simulink model "untitled"  (R2022a)
settings: Solver=FixedStepDiscrete  StartTime=0.0  StopTime=10.0  RelTol=1e-3
libraries: simulink x7
settings Model: DataDictionary=test.sldd  Creator=15801  LastModifiedBy=JSF
settings OptimizationCC: DefaultParameterBehavior=Inlined  EnhancedBackFolding=on  PassReuseOutputArgsAs=Individual arguments  ZeroExternalMemoryAtStartup=off  ZeroInternalMemoryAtStartup=off  OptimizeBlockOrder=speed  DifferentSizesBufferReuse=on  OptimizationCustomize=off  EfficientTunableParamExpr=on
settings DebuggingCC: ParameterTunabilityLossMsg=error
settings ModelReferenceCC: EnableRefExpFcnMdlSchedulingChecks=off
settings SFSimCC: MATLABDynamicMemAlloc=off
settings RTWCC: SystemTargetFile=ert.tlc  TemplateMakefile=ert_default_tmf
settings CodeAppCC: ForceParamTrailComments=on  IgnoreCustomStorageClasses=off  OperatorAnnotations=on  SimulinkDataObjDesc=on  SFDataObjDesc=on  InsertBlockDesc=on
settings ERTTargetCC: TargetLangStandard=C99 (ISO)  GenerateSampleERTMain=on  InlinedParameterPlacement=NonHierarchical  ERTCustomFileTemplate=example_file_process.tlc

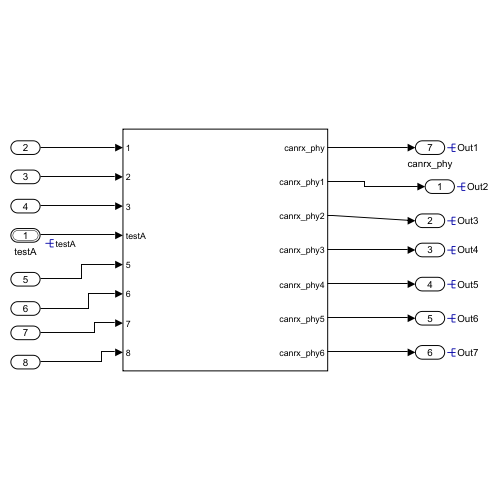
[thumbnail: Simulink's stored preview of the top-level diagram]
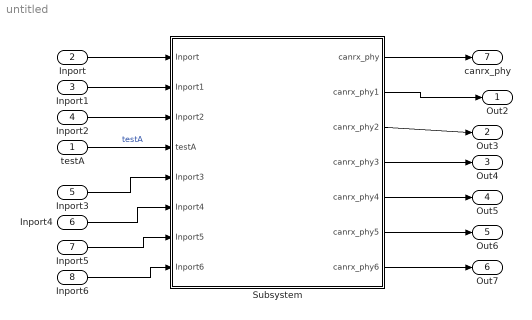
== system untitled ==
  testA : Inport  OutDataTypeStr=Bus: test
  Inport : Inport  Port=2
  Inport1 : Inport  Port=3
  Inport2 : Inport  Port=4
  Inport3 : Inport  Port=5
  Inport4 : Inport  Port=6
  Inport5 : Inport  Port=7
  Inport6 : Inport  Port=8
  Subsystem : Subsystem
  Out2 : Outport  SignalName=Out2
      settings: MustResolveToSignalObject=on
  Out3 : Outport  Port=2  SignalName=Out3
      settings: MustResolveToSignalObject=on
  Out4 : Outport  Port=3  SignalName=Out4
      settings: MustResolveToSignalObject=on
  Out5 : Outport  Port=4  SignalName=Out5
      settings: MustResolveToSignalObject=on
  Out6 : Outport  Port=5  SignalName=Out6
      settings: MustResolveToSignalObject=on
  Out7 : Outport  Port=6  SignalName=Out7
      settings: MustResolveToSignalObject=on
  canrx_phy : Outport  Port=7  SignalName=Out1
      settings: MustResolveToSignalObject=on
  wires:
  Subsystem/5(canrx_phy4) -> Out5/1
  Inport/1 -> Subsystem/1(Inport)
  Inport1/1 -> Subsystem/2(Inport1)
  Inport6/1 -> Subsystem/8(Inport6)
  testA/1 -> Subsystem/4(testA)  "testA"
  Inport3/1 -> Subsystem/5(Inport3)
  Inport2/1 -> Subsystem/3(Inport2)
  Inport4/1 -> Subsystem/6(Inport4)
  Inport5/1 -> Subsystem/7(Inport5)
  Subsystem/1(canrx_phy) -> canrx_phy/1
  Subsystem/2(canrx_phy1) -> Out2/1
  Subsystem/3(canrx_phy2) -> Out3/1
  Subsystem/4(canrx_phy3) -> Out4/1
  Subsystem/6(canrx_phy5) -> Out6/1
  Subsystem/7(canrx_phy6) -> Out7/1

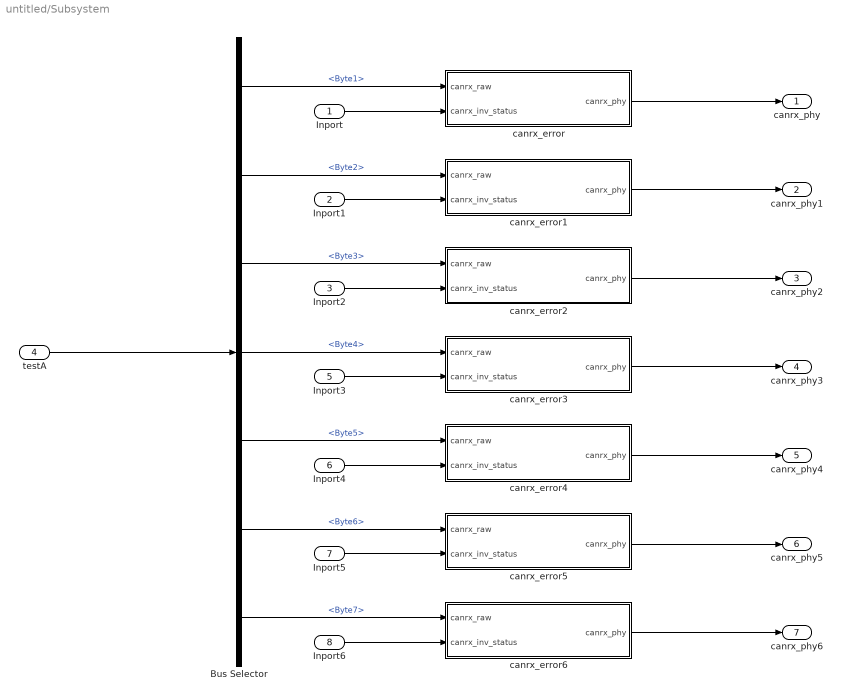
== system untitled/Subsystem ==
  Inport : Inport
  Inport1 : Inport  Port=2
  Inport2 : Inport  Port=3
  testA : Inport  Port=4
  Inport3 : Inport  Port=5
  Inport4 : Inport  Port=6
  Inport5 : Inport  Port=7
  Inport6 : Inport  Port=8
  Bus Selector : BusSelector  OutputSignals=Byte1,Byte2,Byte3,Byte4,Byte5,Byte6,Byte7
  canrx_error : Subsystem  TreatAsAtomicUnit=on
  canrx_error1 : Subsystem  TreatAsAtomicUnit=on
  canrx_error2 : Subsystem  TreatAsAtomicUnit=on
  canrx_error3 : Subsystem  TreatAsAtomicUnit=on
  canrx_error4 : Subsystem  TreatAsAtomicUnit=on
  canrx_error5 : Subsystem  TreatAsAtomicUnit=on
  canrx_error6 : Subsystem  TreatAsAtomicUnit=on
  canrx_phy : Outport
  canrx_phy1 : Outport  Port=2
  canrx_phy2 : Outport  Port=3
  canrx_phy3 : Outport  Port=4
  canrx_phy4 : Outport  Port=5
  canrx_phy5 : Outport  Port=6
  canrx_phy6 : Outport  Port=7
  wires:
  Bus Selector/1 -> canrx_error/1(canrx_raw)  "<Byte1>"
  Bus Selector/2 -> canrx_error1/1(canrx_raw)  "<Byte2>"
  Inport1/1 -> canrx_error1/2(canrx_inv_status)
  Inport/1 -> canrx_error/2(canrx_inv_status)
  Inport6/1 -> canrx_error6/2(canrx_inv_status)
  Bus Selector/7 -> canrx_error6/1(canrx_raw)  "<Byte7>"
  Bus Selector/6 -> canrx_error5/1(canrx_raw)  "<Byte6>"
  Inport2/1 -> canrx_error2/2(canrx_inv_status)
  canrx_error5/1(canrx_phy) -> canrx_phy5/1
  Inport5/1 -> canrx_error5/2(canrx_inv_status)
  Bus Selector/3 -> canrx_error2/1(canrx_raw)  "<Byte3>"
  Bus Selector/5 -> canrx_error4/1(canrx_raw)  "<Byte5>"
  Bus Selector/4 -> canrx_error3/1(canrx_raw)  "<Byte4>"
  Inport3/1 -> canrx_error3/2(canrx_inv_status)
  Inport4/1 -> canrx_error4/2(canrx_inv_status)
  canrx_error6/1(canrx_phy) -> canrx_phy6/1
  testA/1 -> Bus Selector/1
  canrx_error3/1(canrx_phy) -> canrx_phy3/1
  canrx_error/1(canrx_phy) -> canrx_phy/1
  canrx_error4/1(canrx_phy) -> canrx_phy4/1
  canrx_error1/1(canrx_phy) -> canrx_phy1/1
  canrx_error2/1(canrx_phy) -> canrx_phy2/1

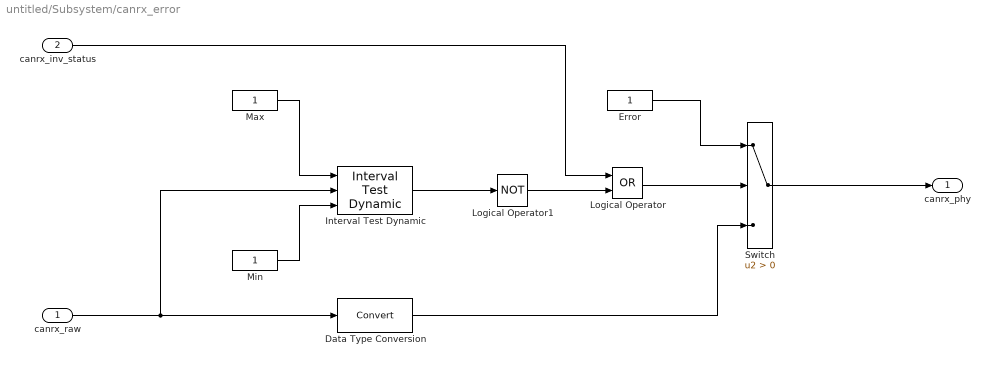
== system untitled/Subsystem/canrx_error ==
  canrx_raw : Inport
  canrx_inv_status : Inport  Port=2
  Data Type Conversion : DataTypeConversion  SaturateOnIntegerOverflow=off  RndMeth=Floor
  Error : Constant  OutDataTypeStr=Inherit: Inherit via back propagation
  Interval Test Dynamic : simulink/Logic and Bit Operations/Interval Test Dynamic  IntervalClosedRight=on  IntervalClosedLeft=on  OutDataTypeStr=boolean
  Logical Operator : Logic  Operator=OR  AllPortsSameDT=off  OutDataTypeStr=boolean
  Logical Operator1 : Logic  Operator=NOT  AllPortsSameDT=off  OutDataTypeStr=boolean
  Max : Constant  OutDataTypeStr=Inherit: Inherit via back propagation
  Min : Constant  OutDataTypeStr=Inherit: Inherit via back propagation
  Switch : Switch  Criteria=u2 > Threshold  SaturateOnIntegerOverflow=off  InputSameDT=off
  canrx_phy : Outport
  wires:
  canrx_raw/1 -> Data Type Conversion/1, Interval Test Dynamic/2
  Max/1 -> Interval Test Dynamic/1
  Min/1 -> Interval Test Dynamic/3
  Data Type Conversion/1 -> Switch/3
  Interval Test Dynamic/1 -> Logical Operator1/1
  Logical Operator1/1 -> Logical Operator/2
  canrx_inv_status/1 -> Logical Operator/1
  Logical Operator/1 -> Switch/2
  Error/1 -> Switch/1
  Switch/1 -> canrx_phy/1

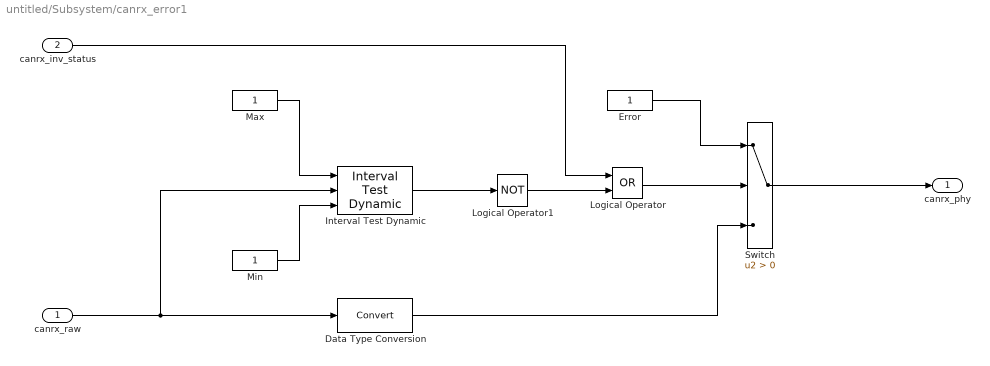
== system untitled/Subsystem/canrx_error1 ==
  canrx_raw : Inport
  canrx_inv_status : Inport  Port=2
  Data Type Conversion : DataTypeConversion  SaturateOnIntegerOverflow=off  RndMeth=Floor
  Error : Constant  OutDataTypeStr=Inherit: Inherit via back propagation
  Interval Test Dynamic : simulink/Logic and Bit Operations/Interval Test Dynamic  IntervalClosedRight=on  IntervalClosedLeft=on  OutDataTypeStr=boolean
  Logical Operator : Logic  Operator=OR  AllPortsSameDT=off  OutDataTypeStr=boolean
  Logical Operator1 : Logic  Operator=NOT  AllPortsSameDT=off  OutDataTypeStr=boolean
  Max : Constant  OutDataTypeStr=Inherit: Inherit via back propagation
  Min : Constant  OutDataTypeStr=Inherit: Inherit via back propagation
  Switch : Switch  Criteria=u2 > Threshold  SaturateOnIntegerOverflow=off  InputSameDT=off
  canrx_phy : Outport
  wires:
  canrx_raw/1 -> Data Type Conversion/1, Interval Test Dynamic/2
  Max/1 -> Interval Test Dynamic/1
  Min/1 -> Interval Test Dynamic/3
  Data Type Conversion/1 -> Switch/3
  Interval Test Dynamic/1 -> Logical Operator1/1
  Logical Operator1/1 -> Logical Operator/2
  canrx_inv_status/1 -> Logical Operator/1
  Logical Operator/1 -> Switch/2
  Error/1 -> Switch/1
  Switch/1 -> canrx_phy/1

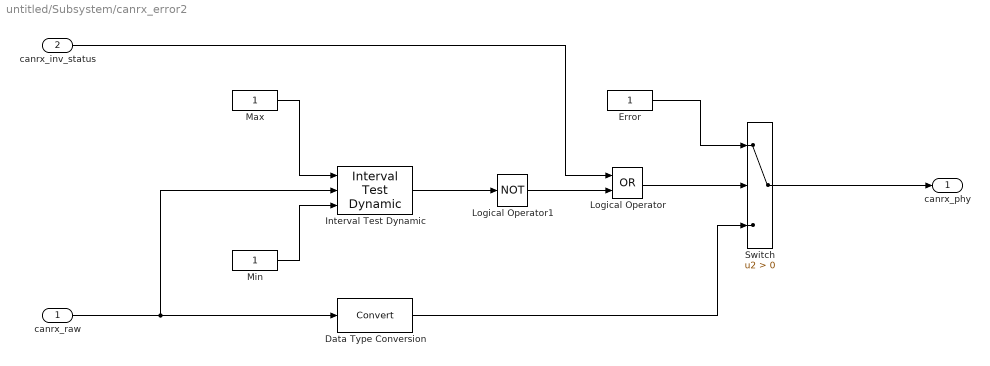
== system untitled/Subsystem/canrx_error2 ==
  canrx_raw : Inport
  canrx_inv_status : Inport  Port=2
  Data Type Conversion : DataTypeConversion  SaturateOnIntegerOverflow=off  RndMeth=Floor
  Error : Constant  OutDataTypeStr=Inherit: Inherit via back propagation
  Interval Test Dynamic : simulink/Logic and Bit Operations/Interval Test Dynamic  IntervalClosedRight=on  IntervalClosedLeft=on  OutDataTypeStr=boolean
  Logical Operator : Logic  Operator=OR  AllPortsSameDT=off  OutDataTypeStr=boolean
  Logical Operator1 : Logic  Operator=NOT  AllPortsSameDT=off  OutDataTypeStr=boolean
  Max : Constant  OutDataTypeStr=Inherit: Inherit via back propagation
  Min : Constant  OutDataTypeStr=Inherit: Inherit via back propagation
  Switch : Switch  Criteria=u2 > Threshold  SaturateOnIntegerOverflow=off  InputSameDT=off
  canrx_phy : Outport
  wires:
  canrx_raw/1 -> Data Type Conversion/1, Interval Test Dynamic/2
  Max/1 -> Interval Test Dynamic/1
  Min/1 -> Interval Test Dynamic/3
  Data Type Conversion/1 -> Switch/3
  Interval Test Dynamic/1 -> Logical Operator1/1
  Logical Operator1/1 -> Logical Operator/2
  canrx_inv_status/1 -> Logical Operator/1
  Logical Operator/1 -> Switch/2
  Error/1 -> Switch/1
  Switch/1 -> canrx_phy/1

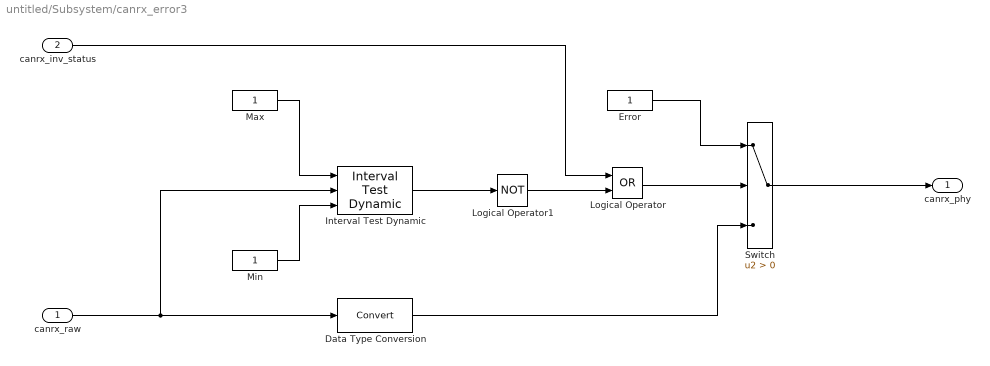
== system untitled/Subsystem/canrx_error3 ==
  canrx_raw : Inport
  canrx_inv_status : Inport  Port=2
  Data Type Conversion : DataTypeConversion  SaturateOnIntegerOverflow=off  RndMeth=Floor
  Error : Constant  OutDataTypeStr=Inherit: Inherit via back propagation
  Interval Test Dynamic : simulink/Logic and Bit Operations/Interval Test Dynamic  IntervalClosedRight=on  IntervalClosedLeft=on  OutDataTypeStr=boolean
  Logical Operator : Logic  Operator=OR  AllPortsSameDT=off  OutDataTypeStr=boolean
  Logical Operator1 : Logic  Operator=NOT  AllPortsSameDT=off  OutDataTypeStr=boolean
  Max : Constant  OutDataTypeStr=Inherit: Inherit via back propagation
  Min : Constant  OutDataTypeStr=Inherit: Inherit via back propagation
  Switch : Switch  Criteria=u2 > Threshold  SaturateOnIntegerOverflow=off  InputSameDT=off
  canrx_phy : Outport
  wires:
  canrx_raw/1 -> Data Type Conversion/1, Interval Test Dynamic/2
  Max/1 -> Interval Test Dynamic/1
  Min/1 -> Interval Test Dynamic/3
  Data Type Conversion/1 -> Switch/3
  Interval Test Dynamic/1 -> Logical Operator1/1
  Logical Operator1/1 -> Logical Operator/2
  canrx_inv_status/1 -> Logical Operator/1
  Logical Operator/1 -> Switch/2
  Error/1 -> Switch/1
  Switch/1 -> canrx_phy/1

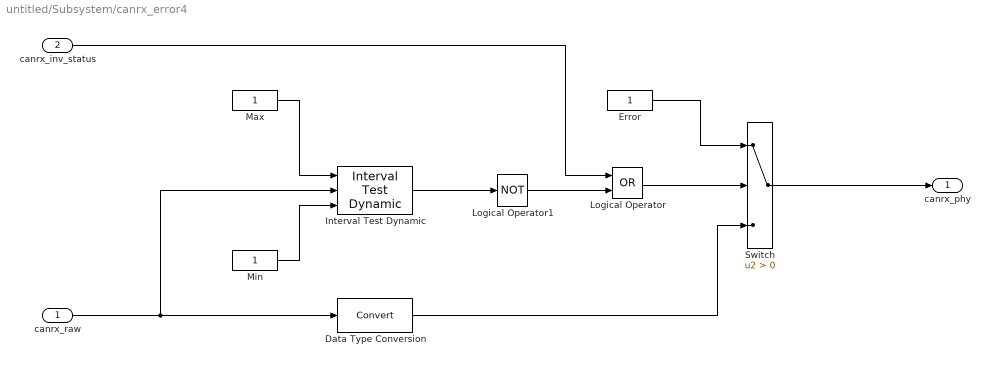
== system untitled/Subsystem/canrx_error4 ==
  canrx_raw : Inport
  canrx_inv_status : Inport  Port=2
  Data Type Conversion : DataTypeConversion  SaturateOnIntegerOverflow=off  RndMeth=Floor
  Error : Constant  OutDataTypeStr=Inherit: Inherit via back propagation
  Interval Test Dynamic : simulink/Logic and Bit Operations/Interval Test Dynamic  IntervalClosedRight=on  IntervalClosedLeft=on  OutDataTypeStr=boolean
  Logical Operator : Logic  Operator=OR  AllPortsSameDT=off  OutDataTypeStr=boolean
  Logical Operator1 : Logic  Operator=NOT  AllPortsSameDT=off  OutDataTypeStr=boolean
  Max : Constant  OutDataTypeStr=Inherit: Inherit via back propagation
  Min : Constant  OutDataTypeStr=Inherit: Inherit via back propagation
  Switch : Switch  Criteria=u2 > Threshold  SaturateOnIntegerOverflow=off  InputSameDT=off
  canrx_phy : Outport
  wires:
  canrx_raw/1 -> Data Type Conversion/1, Interval Test Dynamic/2
  Max/1 -> Interval Test Dynamic/1
  Min/1 -> Interval Test Dynamic/3
  Data Type Conversion/1 -> Switch/3
  Interval Test Dynamic/1 -> Logical Operator1/1
  Logical Operator1/1 -> Logical Operator/2
  canrx_inv_status/1 -> Logical Operator/1
  Logical Operator/1 -> Switch/2
  Error/1 -> Switch/1
  Switch/1 -> canrx_phy/1

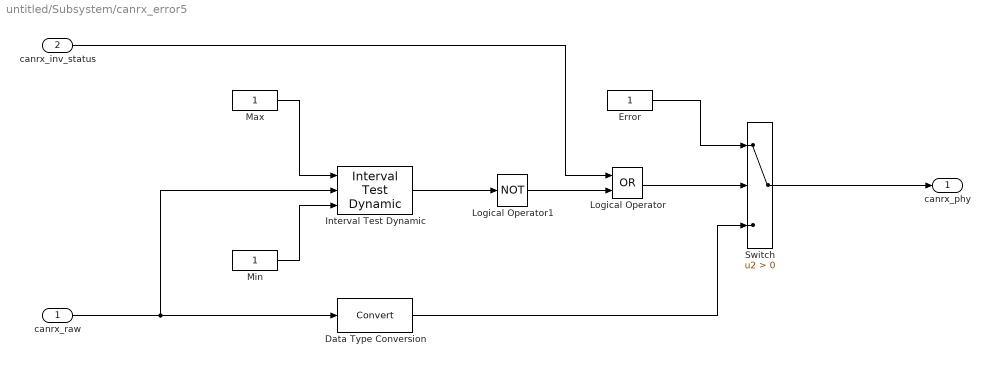
== system untitled/Subsystem/canrx_error5 ==
  canrx_raw : Inport
  canrx_inv_status : Inport  Port=2
  Data Type Conversion : DataTypeConversion  SaturateOnIntegerOverflow=off  RndMeth=Floor
  Error : Constant  OutDataTypeStr=Inherit: Inherit via back propagation
  Interval Test Dynamic : simulink/Logic and Bit Operations/Interval Test Dynamic  IntervalClosedRight=on  IntervalClosedLeft=on  OutDataTypeStr=boolean
  Logical Operator : Logic  Operator=OR  AllPortsSameDT=off  OutDataTypeStr=boolean
  Logical Operator1 : Logic  Operator=NOT  AllPortsSameDT=off  OutDataTypeStr=boolean
  Max : Constant  OutDataTypeStr=Inherit: Inherit via back propagation
  Min : Constant  OutDataTypeStr=Inherit: Inherit via back propagation
  Switch : Switch  Criteria=u2 > Threshold  SaturateOnIntegerOverflow=off  InputSameDT=off
  canrx_phy : Outport
  wires:
  canrx_raw/1 -> Data Type Conversion/1, Interval Test Dynamic/2
  Max/1 -> Interval Test Dynamic/1
  Min/1 -> Interval Test Dynamic/3
  Data Type Conversion/1 -> Switch/3
  Interval Test Dynamic/1 -> Logical Operator1/1
  Logical Operator1/1 -> Logical Operator/2
  canrx_inv_status/1 -> Logical Operator/1
  Logical Operator/1 -> Switch/2
  Error/1 -> Switch/1
  Switch/1 -> canrx_phy/1

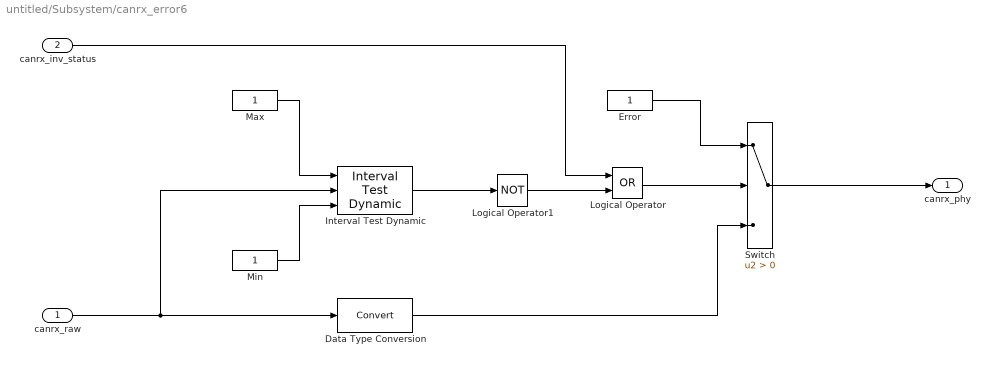
== system untitled/Subsystem/canrx_error6 ==
  canrx_raw : Inport
  canrx_inv_status : Inport  Port=2
  Data Type Conversion : DataTypeConversion  SaturateOnIntegerOverflow=off  RndMeth=Floor
  Error : Constant  OutDataTypeStr=Inherit: Inherit via back propagation
  Interval Test Dynamic : simulink/Logic and Bit Operations/Interval Test Dynamic  IntervalClosedRight=on  IntervalClosedLeft=on  OutDataTypeStr=boolean
  Logical Operator : Logic  Operator=OR  AllPortsSameDT=off  OutDataTypeStr=boolean
  Logical Operator1 : Logic  Operator=NOT  AllPortsSameDT=off  OutDataTypeStr=boolean
  Max : Constant  OutDataTypeStr=Inherit: Inherit via back propagation
  Min : Constant  OutDataTypeStr=Inherit: Inherit via back propagation
  Switch : Switch  Criteria=u2 > Threshold  SaturateOnIntegerOverflow=off  InputSameDT=off
  canrx_phy : Outport
  wires:
  canrx_raw/1 -> Data Type Conversion/1, Interval Test Dynamic/2
  Max/1 -> Interval Test Dynamic/1
  Min/1 -> Interval Test Dynamic/3
  Data Type Conversion/1 -> Switch/3
  Interval Test Dynamic/1 -> Logical Operator1/1
  Logical Operator1/1 -> Logical Operator/2
  canrx_inv_status/1 -> Logical Operator/1
  Logical Operator/1 -> Switch/2
  Error/1 -> Switch/1
  Switch/1 -> canrx_phy/1
